simulink model "Fm"  (R2020b)
settings: Solver=VariableStepAuto  StartTime=0.0  StopTime=10.0  RelTol=1e-3
settings Model: Creator=mluser  LastModifiedBy=mluser

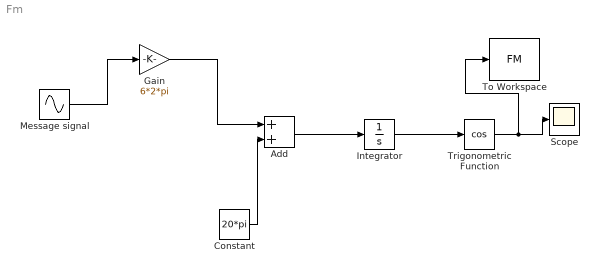
== system Fm ==
  Add : Sum
  Constant : Constant  Value=20*pi
  Gain : Gain  Gain=6*2*pi
  Integrator : Integrator
  Message signal : Sin  Frequency=2*pi  Phase=pi/2  SampleTime=1/5000
  Scope : Scope
  To Workspace : ToWorkspace  VariableName=FM  SampleTime=-1
      settings: Save2DSignal=2-D array (concatenate along first dimension)
  Trigonometric Function : Trigonometry  Operator=cos
  wires:
  Message signal/1 -> Gain/1
  Gain/1 -> Add/1
  Constant/1 -> Add/2
  Add/1 -> Integrator/1
  Integrator/1 -> Trigonometric Function/1
  Trigonometric Function/1 -> To Workspace/1, Scope/1
